simulink model "Sistema_in_catena_aperta"  (R2014a)
settings: Solver=ode45  StartTime=0.0  StopTime=20  RelTol=1e-3
values from neighbouring files (symbols this model uses):
  Ku = 1/dcgain(F1)    [E01.m]
libraries: cstblocks x2
settings Model: Creator=Davide  LastModifiedBy=Davide

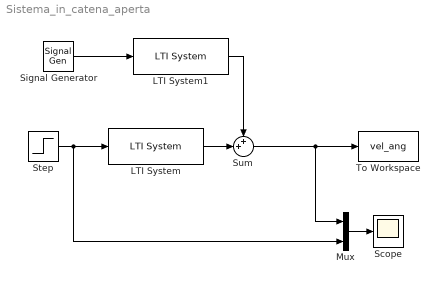
== system Sistema_in_catena_aperta ==
  LTI System : cstblocks/LTI System  sys=F1  IC=[]
  LTI System1 : cstblocks/LTI System  sys=F2  IC=[]
  Mux : Mux  Inputs=2
  Scope : Scope
  Signal Generator : SignalGenerator  WaveForm=square  Amplitude=0.05  Frequency=0.1
  Step : Step  Time=0  After=Ku  SampleTime=0
  Sum : Sum  Inputs=++|
  To Workspace : ToWorkspace  VariableName=vel_ang  SaveFormat=Timeseries  SampleTime=-1
  wires:
  Step/1 -> Mux/2, LTI System/1
  LTI System/1 -> Sum/2
  LTI System1/1 -> Sum/1
  Signal Generator/1 -> LTI System1/1
  Sum/1 -> To Workspace/1, Mux/1
  Mux/1 -> Scope/1
